simulink model "LBR7_Single_TaskComputedTorque"  (R2017b)
settings: Solver=FixedStepAuto  StartTime=0.0  StopTime=12  FixedStep=0.01  RelTol=1e-3
PreLoadFcn:
  | Preload
values from neighbouring files (symbols this model uses):
  cor_gain = -1    [Preload.m]
  joint1_gain = 1    [Preload.m]    (also in PreloadTest.m)
  joint2_gain = 1    [Preload.m]    (also in PreloadTest.m)
  joint3_gain = 1    [Preload.m]    (also in PreloadTest.m)
  joint4_gain = 1    [Preload.m]    (also in PreloadTest.m)
  joint5_gain = 1    [Preload.m]    (also in PreloadTest.m)
  joint6_gain = 1    [Preload.m]    (also in PreloadTest.m)
  joint7_gain = 1    [Preload.m]    (also in PreloadTest.m)
  kuk = SerialLink(L)    [Preload.m]    (also in PreloadTest.m)
undefined symbols (not defined in the file or in its folder): cory, gravy, inertdyn, X, Y, Z
libraries: sm_lib x77, nesl_utility x30
(part 1 of 2)
settings Model: Creator=jrv  LastModifiedBy=jrv

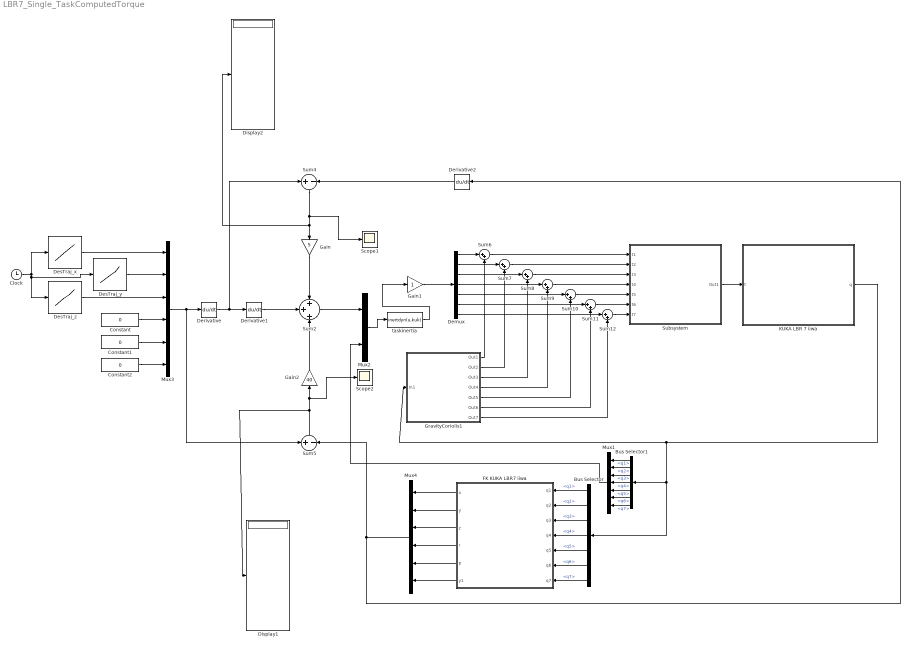
== system LBR7_Single_TaskComputedTorque ==
  Bus Selector : BusSelector  OutputSignals=q1,q2,q3,q4,q5,q6,q7
  Bus Selector1 : BusSelector  OutputSignals=q1,q2,q3,q4,q5,q6,q7
  Clock : Clock
  Constant : Constant  Value=0
  Constant1 : Constant  Value=0
  Constant2 : Constant  Value=0
  Demux : Demux  Outputs=7
  Derivative : Derivative
  Derivative1 : Derivative
  Derivative2 : Derivative
  DesTraj_x : Lookup_n-D  NumberOfTableDimensions=1  BreakpointsForDimension1=[0 5]  Table=[0.2314 0.2314]  ExtrapMethod=Clip  UseLastTableValue=on  InternalRulePriority=Speed  RndMeth=Simplest  InputSameDT=on
  DesTraj_y : Lookup_n-D  NumberOfTableDimensions=1  BreakpointsForDimension1=[0 12]  Table=[-0.2689 0.0689]  ExtrapMethod=Clip  UseLastTableValue=on  InternalRulePriority=Speed  RndMeth=Simplest  InputSameDT=on
  DesTraj_z : Lookup_n-D  NumberOfTableDimensions=1  BreakpointsForDimension1=[0 3 6 9 12]  Table=[0.9093 0.7093 0.9093 0.7093 0.9093]  InterpMethod=Cubic spline  ExtrapMethod=Clip  UseLastTableValue=on  InternalRulePriority=Speed  RndMeth=Simplest  InputSameDT=on
  Display1 : Display
  Display2 : Display
  FK KUKA LBR7 iiwa : MATLAB Function  TreatAsAtomicUnit=on
  Gain : Gain  Gain=5
  Gain1 : Gain
  Gain2 : Gain  Gain=40
  GravityCoriolis1 : Subsystem
  KUKA LBR 7 iiwa : Subsystem
  Mux1 : Mux  Inputs=7
  Mux2 : Mux  Inputs=2
  Mux3 : Mux  Inputs=6
  Mux4 : Mux  Inputs=6
  Scope1 : Scope
  Scope2 : Scope
  Subsystem : Subsystem
  Sum{6..12} (7 alike) : Sum  Inputs=|++
  Sum2 : Sum  Inputs=+++
  Sum4 : Sum  Inputs=+-
  Sum5 : Sum  Inputs=+-
  taskinertia : MATLABFcn  MATLABFcn=inertdyn(u,kuk)
  wires:
  Subsystem/1(Out1) -> KUKA LBR 7 iiwa/1(t)
  Sum4/1 -> Scope1/1, Display2/1, Gain/1
  Sum5/1 -> Scope2/1, Gain2/1, Display1/1
  GravityCoriolis1/1(Out1) -> Sum6/2
  Sum8/1 -> Subsystem/3(t3)
  GravityCoriolis1/4(Out4) -> Sum9/2
  GravityCoriolis1/2(Out2) -> Sum7/2
  Sum9/1 -> Subsystem/4(t4)
  Sum11/1 -> Subsystem/6(t6)
  Demux/7 -> Sum12/1
  Demux/5 -> Sum10/1
  GravityCoriolis1/5(Out5) -> Sum10/2
  Sum6/1 -> Subsystem/1(t1)
  Demux/1 -> Sum6/1
  Sum10/1 -> Subsystem/5(t5)
  Demux/6 -> Sum11/1
  Demux/3 -> Sum8/1
  GravityCoriolis1/6(Out6) -> Sum11/2
  Demux/4 -> Sum9/1
  Demux/2 -> Sum7/1
  Sum7/1 -> Subsystem/2(t2)
  GravityCoriolis1/3(Out3) -> Sum8/2
  Sum12/1 -> Subsystem/7(t7)
  GravityCoriolis1/7(Out7) -> Sum12/2
  Gain/1 -> Sum2/1
  Gain2/1 -> Sum2/3
  DesTraj_x/1 -> Mux3/1
  Constant2/1 -> Mux3/6
  DesTraj_y/1 -> Mux3/2
  Constant/1 -> Mux3/4
  Clock/1 -> DesTraj_y/1, DesTraj_z/1, DesTraj_x/1
  Constant1/1 -> Mux3/5
  DesTraj_z/1 -> Mux3/3
  Mux3/1 -> Sum5/1, Derivative/1
  Derivative/1 -> Sum4/1, Derivative1/1
  Derivative1/1 -> Sum2/2
  Bus Selector/1 -> FK KUKA LBR7 iiwa/1(q1)  "<q1>"
  Bus Selector/3 -> FK KUKA LBR7 iiwa/3(q3)  "<q3>"
  Bus Selector/5 -> FK KUKA LBR7 iiwa/5(q5)  "<q5>"
  Bus Selector/6 -> FK KUKA LBR7 iiwa/6(q6)  "<q6>"
  Bus Selector/2 -> FK KUKA LBR7 iiwa/2(q2)  "<q2>"
  Bus Selector/7 -> FK KUKA LBR7 iiwa/7(q7)  "<q7>"
  Bus Selector/4 -> FK KUKA LBR7 iiwa/4(q4)  "<q4>"
  FK KUKA LBR7 iiwa/3(z) -> Mux4/3
  FK KUKA LBR7 iiwa/2(y) -> Mux4/2
  FK KUKA LBR7 iiwa/4(r) -> Mux4/4
  FK KUKA LBR7 iiwa/1(x) -> Mux4/1
  FK KUKA LBR7 iiwa/5(p) -> Mux4/5
  FK KUKA LBR7 iiwa/6(y1) -> Mux4/6
  Mux4/1 -> Sum5/2, Derivative2/1
  Mux2/1 -> taskinertia/1
  taskinertia/1 -> Gain1/1
  Sum2/1 -> Mux2/1
  Mux1/1 -> Mux2/2
  KUKA LBR 7 iiwa/1(q) -> GravityCoriolis1/1(In1), Bus Selector1/1, Bus Selector/1
  Bus Selector1/1 -> Mux1/1  "<q1>"
  Bus Selector1/2 -> Mux1/2  "<q2>"
  Bus Selector1/3 -> Mux1/3  "<q3>"
  Bus Selector1/4 -> Mux1/4  "<q4>"
  Bus Selector1/5 -> Mux1/5  "<q5>"
  Bus Selector1/6 -> Mux1/6  "<q6>"
  Bus Selector1/7 -> Mux1/7  "<q7>"
  Derivative2/1 -> Sum4/2
  Gain1/1 -> Demux/1

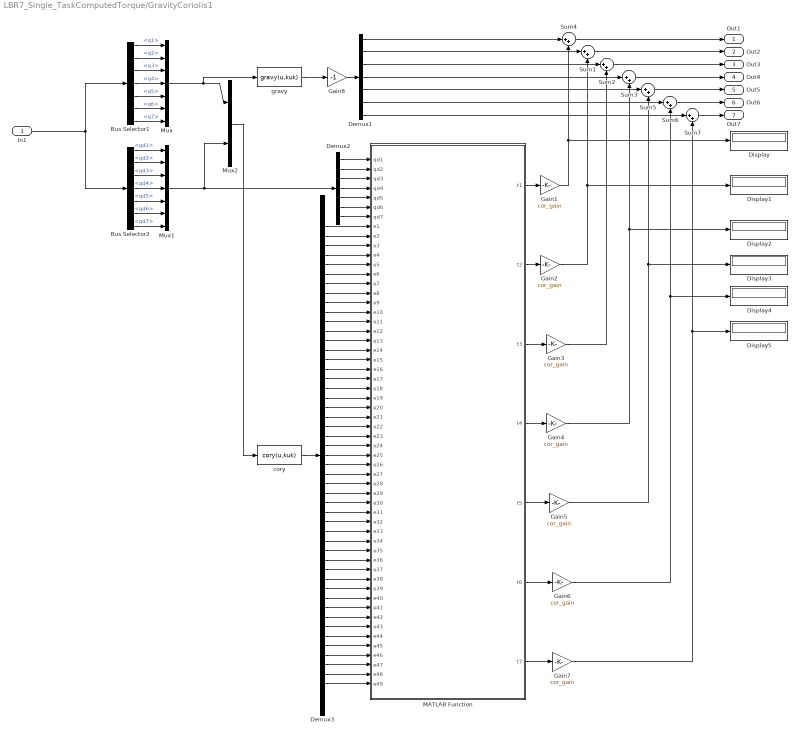
== system LBR7_Single_TaskComputedTorque/GravityCoriolis1 ==
  In1 : Inport
  Bus Selector1 : BusSelector  OutputSignals=q1,q2,q3,q4,q5,q6,q7
  Bus Selector2 : BusSelector  OutputSignals=qd1,qd2,qd3,qd4,qd5,qd6,qd7
  Demux1 : Demux  Outputs=7
  Demux2 : Demux  Outputs=7
  Demux3 : Demux  Outputs=49
  Display{,1..5} (6 alike) : Display
  Gain{1..7} (7 alike) : Gain  Gain=cor_gain
  Gain8 : Gain  Gain=-1
  MATLAB Function : MATLAB Function  TreatAsAtomicUnit=on
  Mux : Mux  Inputs=7
  Mux1 : Mux  Inputs=7
  Mux2 : Mux  Inputs=2
  Sum{1..7} (7 alike) : Sum  Inputs=|++
  cory : MATLABFcn  MATLABFcn=cory(u,kuk)
  gravy : MATLABFcn  MATLABFcn=gravy(u,kuk)
  Out1 : Outport
  Out2 : Outport  Port=2
  Out3 : Outport  Port=3
  Out4 : Outport  Port=4
  Out5 : Outport  Port=5
  Out6 : Outport  Port=6
  Out7 : Outport  Port=7
  wires:
  Demux2/1 -> MATLAB Function/1(qd1)
  Mux1/1 -> Mux2/2, Demux2/1
  Demux3/16 -> MATLAB Function/23(e16)
  Mux/1 -> gravy/1, Mux2/1
  Bus Selector1/2 -> Mux/2  "<q2>"
  Demux3/29 -> MATLAB Function/36(e29)
  Demux3/35 -> MATLAB Function/42(e35)
  Demux3/15 -> MATLAB Function/22(e15)
  Demux3/22 -> MATLAB Function/29(e22)
  Demux3/9 -> MATLAB Function/16(e9)
  Bus Selector1/3 -> Mux/3  "<q3>"
  Demux3/11 -> MATLAB Function/18(e11)
  Bus Selector1/7 -> Mux/7  "<q7>"
  Demux3/42 -> MATLAB Function/49(e42)
  Demux3/43 -> MATLAB Function/50(e43)
  Bus Selector1/1 -> Mux/1  "<q1>"
  Bus Selector1/5 -> Mux/5  "<q5>"
  Demux3/24 -> MATLAB Function/31(e24)
  Bus Selector1/6 -> Mux/6  "<q6>"
  Demux3/26 -> MATLAB Function/33(e26)
  Bus Selector1/4 -> Mux/4  "<q4>"
  Demux3/14 -> MATLAB Function/21(e14)
  Demux3/19 -> MATLAB Function/26(e19)
  Demux3/4 -> MATLAB Function/11(e4)
  Bus Selector2/4 -> Mux1/4  "<qd4>"
  cory/1 -> Demux3/1
  Demux3/23 -> MATLAB Function/30(e23)
  Demux2/3 -> MATLAB Function/3(qd3)
  Demux3/31 -> MATLAB Function/38(e31)
  Demux2/4 -> MATLAB Function/4(qd4)
  Demux3/17 -> MATLAB Function/24(e17)
  Demux2/5 -> MATLAB Function/5(qd5)
  Demux3/3 -> MATLAB Function/10(e3)
  Demux3/20 -> MATLAB Function/27(e20)
  Demux3/36 -> MATLAB Function/43(e36)
  In1/1 -> Bus Selector2/1, Bus Selector1/1
  Bus Selector2/6 -> Mux1/6  "<qd6>"
  Demux3/40 -> MATLAB Function/47(e40)
  Demux3/8 -> MATLAB Function/15(e8)
  Demux3/45 -> MATLAB Function/52(e45)
  Demux3/28 -> MATLAB Function/35(e28)
  Demux3/41 -> MATLAB Function/48(e41)
  Bus Selector2/5 -> Mux1/5  "<qd5>"
  Demux3/49 -> MATLAB Function/56(e49)
  Demux3/27 -> MATLAB Function/34(e27)
  Demux3/13 -> MATLAB Function/20(e13)
  Demux3/6 -> MATLAB Function/13(e6)
  Demux3/30 -> MATLAB Function/37(e30)
  Demux2/7 -> MATLAB Function/7(qd7)
  Demux3/25 -> MATLAB Function/32(e25)
  Demux2/2 -> MATLAB Function/2(qd2)
  Demux3/5 -> MATLAB Function/12(e5)
  Bus Selector2/7 -> Mux1/7  "<qd7>"
  Demux3/7 -> MATLAB Function/14(e7)
  Bus Selector2/3 -> Mux1/3  "<qd3>"
  Mux2/1 -> cory/1
  Demux1/1 -> Sum4/1
  Demux3/1 -> MATLAB Function/8(e1)
  Demux3/33 -> MATLAB Function/40(e33)
  Demux3/12 -> MATLAB Function/19(e12)
  Bus Selector2/1 -> Mux1/1  "<qd1>"
  Demux1/4 -> Sum3/1
  Demux3/48 -> MATLAB Function/55(e48)
  Demux3/32 -> MATLAB Function/39(e32)
  Demux3/34 -> MATLAB Function/41(e34)
  Demux3/47 -> MATLAB Function/54(e47)
  Bus Selector2/2 -> Mux1/2  "<qd2>"
  Demux2/6 -> MATLAB Function/6(qd6)
  Sum7/1 -> Out7/1
  Demux3/39 -> MATLAB Function/46(e39)
  Sum3/1 -> Out4/1
  Sum6/1 -> Out6/1
  Demux1/3 -> Sum2/1
  Demux3/21 -> MATLAB Function/28(e21)
  Sum1/1 -> Out2/1
  Demux1/2 -> Sum1/1
  Sum4/1 -> Out1/1
  Demux1/5 -> Sum5/1
  Demux3/2 -> MATLAB Function/9(e2)
  Demux3/18 -> MATLAB Function/25(e18)
  Demux3/38 -> MATLAB Function/45(e38)
  Demux3/46 -> MATLAB Function/53(e46)
  Sum5/1 -> Out5/1
  Demux3/37 -> MATLAB Function/44(e37)
  Demux3/44 -> MATLAB Function/51(e44)
  Sum2/1 -> Out3/1
  Demux3/10 -> MATLAB Function/17(e10)
  Gain2/1 -> Display1/1, Sum1/2
  Gain4/1 -> Display2/1, Sum3/2
  Gain6/1 -> Display4/1, Sum6/2
  Gain3/1 -> Sum2/2
  Gain5/1 -> Display3/1, Sum5/2
  Demux1/7 -> Sum7/1
  Gain7/1 -> Display5/1, Sum7/2
  Gain8/1 -> Demux1/1
  Demux1/6 -> Sum6/1
  gravy/1 -> Gain8/1
  Gain1/1 -> Display/1, Sum4/2
  MATLAB Function/1(t1) -> Gain1/1
  MATLAB Function/2(t2) -> Gain2/1
  MATLAB Function/3(t3) -> Gain3/1
  MATLAB Function/4(t4) -> Gain4/1
  MATLAB Function/5(t5) -> Gain5/1
  MATLAB Function/6(t6) -> Gain6/1
  MATLAB Function/7(t7) -> Gain7/1

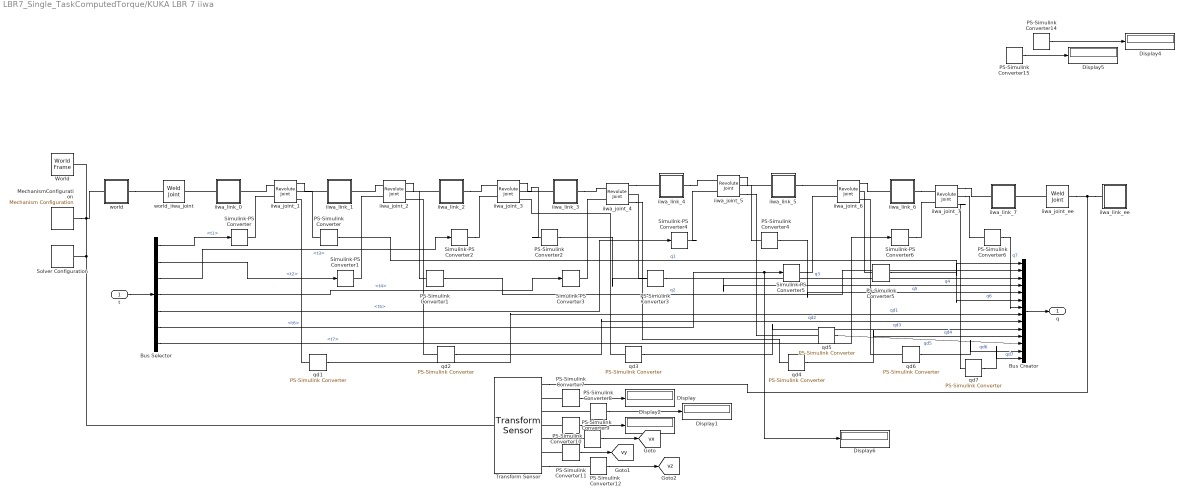
== system LBR7_Single_TaskComputedTorque/KUKA LBR 7 iiwa ==
  t : Inport
  Bus Creator : BusCreator  Inputs=14
  Bus Selector : BusSelector  OutputSignals=t1,t2,t3,t4,t5,t6,t7
  Display{,1..2,4..6} (6 alike) : Display
  MechanismConfiguration : sm_lib/Utilities/Mechanism Configuration  UniformGravity=Constant  GravityVector=[0 0 -9.81]  GravityUnits=m/s^2  LinearizationDelta=0.001
  PS-Simulink Converter{,1..6} (7 alike) : nesl_utility/PS-Simulink Converter  PhysicalDomain=network_engine_domain  SubClassName=ps_output  LeftPortType=input  RightPortType=output  PseudoPeriodic=off  Frequencies=[]  Unit=rad  AffineConversion=off
  PS-Simulink Converter10 : nesl_utility/PS-Simulink Converter  PhysicalDomain=network_engine_domain  SubClassName=ps_output  LeftPortType=input  RightPortType=output  PseudoPeriodic=off  Frequencies=[]  Unit=m/s  AffineConversion=off
  PS-Simulink Converter11 : nesl_utility/PS-Simulink Converter  PhysicalDomain=network_engine_domain  SubClassName=ps_output  LeftPortType=input  RightPortType=output  PseudoPeriodic=off  Frequencies=[]  Unit=m/s  AffineConversion=off
  PS-Simulink Converter12 : nesl_utility/PS-Simulink Converter  PhysicalDomain=network_engine_domain  SubClassName=ps_output  LeftPortType=input  RightPortType=output  PseudoPeriodic=off  Frequencies=[]  Unit=m/s  AffineConversion=off
  PS-Simulink Converter{7..9,14..15} (5 alike) : nesl_utility/PS-Simulink Converter  PhysicalDomain=network_engine_domain  SubClassName=ps_output  LeftPortType=input  RightPortType=output  PseudoPeriodic=off  Frequencies=[]  Unit=1  AffineConversion=off
  Simulink-PS Converter{,1..6} (7 alike) : nesl_utility/Simulink-PS Converter  PhysicalDomain=network_engine_domain  SubClassName=ps_input  LeftPortType=input  RightPortType=output  PseudoPeriodic=off  Frequencies=[]  NoiseDistribution=none  NoiseParameters=[]  Unit=N*m  AffineConversion=off  FilteringAndDerivatives=provide  SimscapeFilterOrder=1  InputFilterTimeConstant=0.001  UdotUserProvided=0
  Solver Configuration : nesl_utility/Solver Configuration  PhysicalDomain=network_engine_domain  SubClassName=solver  LeftPortType=input  RightPortType=generic  Accelerate=off  Tones=[]  Harmonics=[]  SimulateNoise=off  Profile=off  UseLocalSampling=off  EnableSwitchedLinearOptims=on  FrequencyDomain=off  UseCCode=off  RelTol=0.001  AbsTol=1e-06  MinStep=1e-09  ToWorkspace=off  RevertToSquareIcSolve=off  NumHomotopyIterations=100  PhasorMode=off  PhasorModeNumHarmonics=1  DoDC=off  ResidualTolerance=1e-09  UseLocalSolver=off  LocalSolverChoice=NE_BACKWARD_EULER_ADVANCER  LocalSolverSampleTime=0.001  DoFixedCost=off  MaxNonlinIter=3  MaxModeIter=2  LinearAlgebra=Sparse  DelaysMemoryBudget=1024  AutomaticFiltering=on  FilteringTimeConstant=0.001
  Transform Sensor : sm_lib/Frames and Transforms/Transform Sensor  MeasurementFrame=World  SenseAngle=off  SenseAxis=off  SenseAngle1=off  SenseAngle2=off  SenseAngle3=off  SenseQ=off  SenseR=off  SenseOmegaX=off  SenseOmegaY=off  SenseOmegaZ=off  SenseOmega1=off  SenseOmega2=off  SenseOmega3=off  SenseQDot=off  SenseRDot=off  SenseAlphaX=off  SenseAlphaY=off  SenseAlphaZ=off  SenseAlpha1=off  SenseAlpha2=off  SenseAlpha3=off  SenseQDDot=off  SenseRDDot=off  SenseX=on  SenseY=on  SenseZ=on  SenseRad=off  SenseAzim=off  SenseDist=off  SenseInc=off  SenseXDot=on  SenseYDot=on  SenseZDot=on  SenseRadDot=off  SenseAzimDot=off  SenseDistDot=off  SenseIncDot=off  SenseXDDot=off  SenseYDDot=off  SenseZDDot=off  SenseRadDDot=off  SenseAzimDDot=off  SenseDistDDot=off  SenseIncDDot=off
  World : sm_lib/Frames and Transforms/World Frame
  iiwa_joint_1 : sm_lib/Joints/Revolute Joint  SenseConstraintForce=off  SenseConstraintForceX=off  SenseConstraintForceY=off  SenseConstraintForceZ=off  SenseConstraintTorque=off  SenseConstraintTorqueX=off  SenseConstraintTorqueY=off  SenseConstraintTorqueZ=off  SenseTotalForce=off  SenseTotalForceX=off  SenseTotalForceY=off  SenseTotalForceZ=off  SenseTotalTorque=off  SenseTotalTorqueX=off  SenseTotalTorqueY=off  SenseTotalTorqueZ=off  CompositeWrenchDir=FollowerOnBase  CompositeWrenchFrame=BaseFrame  EquilibriumPosition=0  EquilibriumPositionUnits=deg  SpringStiffness=0  SpringStiffnessUnits=N*m/deg  DampingCoefficient=joint1_damping  DampingCoefficientUnits=m^2*kg/s/rad  TorqueActuationMode=InputTorque  MotionActuationMode=ComputedMotion  SensePosition=on  SenseVelocity=on  SenseAcceleration=off  SenseTorqueForce=off  PositionTargetSpecify=on  PositionTargetPriority=High  PositionTargetValue=joint1_initial_deg  PositionTargetValueUnits=deg  VelocityTargetSpecify=off  VelocityTargetPriority=High  VelocityTargetValue=0  VelocityTargetValueUnits=deg/s
  iiwa_joint_2 : sm_lib/Joints/Revolute Joint  SenseConstraintForce=off  SenseConstraintForceX=off  SenseConstraintForceY=off  SenseConstraintForceZ=off  SenseConstraintTorque=off  SenseConstraintTorqueX=off  SenseConstraintTorqueY=off  SenseConstraintTorqueZ=off  SenseTotalForce=off  SenseTotalForceX=off  SenseTotalForceY=off  SenseTotalForceZ=off  SenseTotalTorque=off  SenseTotalTorqueX=off  SenseTotalTorqueY=off  SenseTotalTorqueZ=off  CompositeWrenchDir=FollowerOnBase  CompositeWrenchFrame=BaseFrame  EquilibriumPosition=0  EquilibriumPositionUnits=deg  SpringStiffness=0  SpringStiffnessUnits=N*m/deg  DampingCoefficient=joint2_damping  DampingCoefficientUnits=m^2*kg/s/rad  TorqueActuationMode=InputTorque  MotionActuationMode=ComputedMotion  SensePosition=on  SenseVelocity=on  SenseAcceleration=off  SenseTorqueForce=off  PositionTargetSpecify=on  PositionTargetPriority=High  PositionTargetValue=joint2_initial_deg  PositionTargetValueUnits=deg  VelocityTargetSpecify=off  VelocityTargetPriority=High  VelocityTargetValue=0  VelocityTargetValueUnits=deg/s
  iiwa_joint_3 : sm_lib/Joints/Revolute Joint  SenseConstraintForce=off  SenseConstraintForceX=off  SenseConstraintForceY=off  SenseConstraintForceZ=off  SenseConstraintTorque=off  SenseConstraintTorqueX=off  SenseConstraintTorqueY=off  SenseConstraintTorqueZ=off  SenseTotalForce=off  SenseTotalForceX=off  SenseTotalForceY=off  SenseTotalForceZ=off  SenseTotalTorque=off  SenseTotalTorqueX=off  SenseTotalTorqueY=off  SenseTotalTorqueZ=off  CompositeWrenchDir=FollowerOnBase  CompositeWrenchFrame=BaseFrame  EquilibriumPosition=0  EquilibriumPositionUnits=deg  SpringStiffness=0  SpringStiffnessUnits=N*m/deg  DampingCoefficient=joint3_damping  DampingCoefficientUnits=m^2*kg/s/rad  TorqueActuationMode=InputTorque  MotionActuationMode=ComputedMotion  SensePosition=on  SenseVelocity=on  SenseAcceleration=off  SenseTorqueForce=off  PositionTargetSpecify=on  PositionTargetPriority=High  PositionTargetValue=joint3_initial_deg  PositionTargetValueUnits=deg  VelocityTargetSpecify=off  VelocityTargetPriority=High  VelocityTargetValue=0  VelocityTargetValueUnits=deg/s
  iiwa_joint_4 : sm_lib/Joints/Revolute Joint  SenseConstraintForce=off  SenseConstraintForceX=off  SenseConstraintForceY=off  SenseConstraintForceZ=off  SenseConstraintTorque=off  SenseConstraintTorqueX=off  SenseConstraintTorqueY=off  SenseConstraintTorqueZ=off  SenseTotalForce=off  SenseTotalForceX=off  SenseTotalForceY=off  SenseTotalForceZ=off  SenseTotalTorque=off  SenseTotalTorqueX=off  SenseTotalTorqueY=off  SenseTotalTorqueZ=off  CompositeWrenchDir=FollowerOnBase  CompositeWrenchFrame=BaseFrame  EquilibriumPosition=0  EquilibriumPositionUnits=deg  SpringStiffness=0  SpringStiffnessUnits=N*m/deg  DampingCoefficient=joint4_damping  DampingCoefficientUnits=m^2*kg/s/rad  TorqueActuationMode=InputTorque  MotionActuationMode=ComputedMotion  SensePosition=on  SenseVelocity=on  SenseAcceleration=off  SenseTorqueForce=off  PositionTargetSpecify=on  PositionTargetPriority=High  PositionTargetValue=joint4_initial_deg  PositionTargetValueUnits=deg  VelocityTargetSpecify=off  VelocityTargetPriority=High  VelocityTargetValue=0  VelocityTargetValueUnits=deg/s
  iiwa_joint_5 : sm_lib/Joints/Revolute Joint  SenseConstraintForce=off  SenseConstraintForceX=off  SenseConstraintForceY=off  SenseConstraintForceZ=off  SenseConstraintTorque=off  SenseConstraintTorqueX=off  SenseConstraintTorqueY=off  SenseConstraintTorqueZ=off  SenseTotalForce=off  SenseTotalForceX=off  SenseTotalForceY=off  SenseTotalForceZ=off  SenseTotalTorque=off  SenseTotalTorqueX=off  SenseTotalTorqueY=off  SenseTotalTorqueZ=off  CompositeWrenchDir=FollowerOnBase  CompositeWrenchFrame=BaseFrame  EquilibriumPosition=0  EquilibriumPositionUnits=deg  SpringStiffness=0  SpringStiffnessUnits=N*m/deg  DampingCoefficient=joint5_damping  DampingCoefficientUnits=m^2*kg/s/rad  TorqueActuationMode=InputTorque  MotionActuationMode=ComputedMotion  SensePosition=on  SenseVelocity=on  SenseAcceleration=off  SenseTorqueForce=off  PositionTargetSpecify=on  PositionTargetPriority=High  PositionTargetValue=joint5_initial_deg  PositionTargetValueUnits=deg  VelocityTargetSpecify=off  VelocityTargetPriority=High  VelocityTargetValue=0  VelocityTargetValueUnits=deg/s
  iiwa_joint_6 : sm_lib/Joints/Revolute Joint  SenseConstraintForce=off  SenseConstraintForceX=off  SenseConstraintForceY=off  SenseConstraintForceZ=off  SenseConstraintTorque=off  SenseConstraintTorqueX=off  SenseConstraintTorqueY=off  SenseConstraintTorqueZ=off  SenseTotalForce=off  SenseTotalForceX=off  SenseTotalForceY=off  SenseTotalForceZ=off  SenseTotalTorque=off  SenseTotalTorqueX=off  SenseTotalTorqueY=off  SenseTotalTorqueZ=off  CompositeWrenchDir=FollowerOnBase  CompositeWrenchFrame=BaseFrame  EquilibriumPosition=0  EquilibriumPositionUnits=deg  SpringStiffness=0  SpringStiffnessUnits=N*m/deg  DampingCoefficient=joint6_damping  DampingCoefficientUnits=m^2*kg/s/rad  TorqueActuationMode=InputTorque  MotionActuationMode=ComputedMotion  SensePosition=on  SenseVelocity=on  SenseAcceleration=off  SenseTorqueForce=off  PositionTargetSpecify=on  PositionTargetPriority=High  PositionTargetValue=joint6_initial_deg  PositionTargetValueUnits=deg  VelocityTargetSpecify=off  VelocityTargetPriority=High  VelocityTargetValue=0  VelocityTargetValueUnits=deg/s
  iiwa_joint_7 : sm_lib/Joints/Revolute Joint  SenseConstraintForce=off  SenseConstraintForceX=off  SenseConstraintForceY=off  SenseConstraintForceZ=off  SenseConstraintTorque=off  SenseConstraintTorqueX=off  SenseConstraintTorqueY=off  SenseConstraintTorqueZ=off  SenseTotalForce=off  SenseTotalForceX=off  SenseTotalForceY=off  SenseTotalForceZ=off  SenseTotalTorque=off  SenseTotalTorqueX=off  SenseTotalTorqueY=off  SenseTotalTorqueZ=off  CompositeWrenchDir=FollowerOnBase  CompositeWrenchFrame=BaseFrame  EquilibriumPosition=0  EquilibriumPositionUnits=deg  SpringStiffness=0  SpringStiffnessUnits=N*m/deg  DampingCoefficient=joint7_damping  DampingCoefficientUnits=m^2*kg/s/rad  TorqueActuationMode=InputTorque  MotionActuationMode=ComputedMotion  SensePosition=on  SenseVelocity=on  SenseAcceleration=off  SenseTorqueForce=off  PositionTargetSpecify=on  PositionTargetPriority=High  PositionTargetValue=joint7_initial_deg  PositionTargetValueUnits=deg  VelocityTargetSpecify=off  VelocityTargetPriority=High  VelocityTargetValue=0  VelocityTargetValueUnits=deg/s
  iiwa_joint_ee : sm_lib/Joints/Weld Joint  SenseConstraintForce=off  SenseConstraintForceX=off  SenseConstraintForceY=off  SenseConstraintForceZ=off  SenseConstraintTorque=off  SenseConstraintTorqueX=off  SenseConstraintTorqueY=off  SenseConstraintTorqueZ=off  SenseTotalForce=off  SenseTotalForceX=off  SenseTotalForceY=off  SenseTotalForceZ=off  SenseTotalTorque=off  SenseTotalTorqueX=off  SenseTotalTorqueY=off  SenseTotalTorqueZ=off  CompositeWrenchDir=FollowerOnBase  CompositeWrenchFrame=BaseFrame
  iiwa_link_0 : Subsystem
  iiwa_link_1 : Subsystem
  iiwa_link_2 : Subsystem
  iiwa_link_3 : Subsystem
  iiwa_link_4 : Subsystem
  iiwa_link_5 : Subsystem
  iiwa_link_6 : Subsystem
  iiwa_link_7 : Subsystem
  iiwa_link_ee : Subsystem
  qd{1..7} (7 alike) : nesl_utility/PS-Simulink Converter  PhysicalDomain=network_engine_domain  SubClassName=ps_output  LeftPortType=input  RightPortType=output  PseudoPeriodic=off  Frequencies=[]  Unit=rad/s  AffineConversion=off
  world : Subsystem
  world_iiwa_joint : sm_lib/Joints/Weld Joint  SenseConstraintForce=off  SenseConstraintForceX=off  SenseConstraintForceY=off  SenseConstraintForceZ=off  SenseConstraintTorque=off  SenseConstraintTorqueX=off  SenseConstraintTorqueY=off  SenseConstraintTorqueZ=off  SenseTotalForce=off  SenseTotalForceX=off  SenseTotalForceY=off  SenseTotalForceZ=off  SenseTotalTorque=off  SenseTotalTorqueX=off  SenseTotalTorqueY=off  SenseTotalTorqueZ=off  CompositeWrenchDir=FollowerOnBase  CompositeWrenchFrame=BaseFrame
  q : Outport
  tag scope: vx=global, vy=global, vz=global
  wires:
  PS-Simulink Converter7/1 -> Display/1
  PS-Simulink Converter9/1 -> Display2/1
  PS-Simulink Converter8/1 -> Display1/1
  PS-Simulink Converter/1 -> Bus Creator/1  "q1"
  PS-Simulink Converter1/1 -> Bus Creator/2  "q2"
  PS-Simulink Converter2/1 -> Bus Creator/3  "q3"
  PS-Simulink Converter3/1 -> Bus Creator/4  "q4"
  PS-Simulink Converter4/1 -> Bus Creator/5  "q5"
  PS-Simulink Converter5/1 -> Bus Creator/6  "q6"
  PS-Simulink Converter6/1 -> Bus Creator/7  "q7"
  Bus Creator/1 -> q/1
  t/1 -> Bus Selector/1
  Bus Selector/1 -> Simulink-PS Converter/1  "<t1>"
  Bus Selector/2 -> Simulink-PS Converter1/1  "<t2>"
  Bus Selector/3 -> Simulink-PS Converter2/1  "<t3>"
  Bus Selector/4 -> Simulink-PS Converter3/1  "<t4>"
  Bus Selector/5 -> Simulink-PS Converter4/1  "<t5>"
  Bus Selector/6 -> Display6/1, Simulink-PS Converter5/1  "<t6>"
  Bus Selector/7 -> Simulink-PS Converter6/1  "<t7>"
  qd1/1 -> Bus Creator/8  "qd1"
  qd2/1 -> Bus Creator/9  "qd2"
  qd3/1 -> Bus Creator/10  "qd3"
  qd4/1 -> Bus Creator/11  "qd4"
  qd5/1 -> Bus Creator/12  "qd5"
  qd6/1 -> Bus Creator/13  "qd6"
  qd7/1 -> Bus Creator/14  "qd7"
  PS-Simulink Converter10/1 -> [vx]
  PS-Simulink Converter11/1 -> [vy]
  PS-Simulink Converter12/1 -> [vz]
  PS-Simulink Converter14/1 -> Display4/1
  PS-Simulink Converter15/1 -> Display5/1
  connections:
  Simulink-PS Converter/RConn1 -- iiwa_joint_1/LConn2
  PS-Simulink Converter/LConn1 -- iiwa_joint_1/RConn2
  iiwa_joint_2/LConn2 -- Simulink-PS Converter1/RConn1
  iiwa_joint_2/RConn2 -- PS-Simulink Converter1/LConn1
  iiwa_joint_1/LConn1 -- iiwa_link_0/RConn1
  iiwa_joint_2/RConn1 -- iiwa_link_2/LConn1
  iiwa_link_0/LConn1 -- world_iiwa_joint/RConn1
  world/RConn1 -- world_iiwa_joint/LConn1
  World/RConn1 -- Transform Sensor/LConn1 -- Solver Configuration/RConn1 -- MechanismConfiguration/RConn1 -- world/LConn1
  iiwa_joint_2/LConn1 -- iiwa_link_1/RConn1
  iiwa_joint_1/RConn1 -- iiwa_link_1/LConn1
  PS-Simulink Converter9/LConn1 -- Transform Sensor/RConn4
  PS-Simulink Converter8/LConn1 -- Transform Sensor/RConn3
  PS-Simulink Converter7/LConn1 -- Transform Sensor/RConn2
  qd1/LConn1 -- iiwa_joint_1/RConn3
  qd2/LConn1 -- iiwa_joint_2/RConn3
  PS-Simulink Converter10/LConn1 -- Transform Sensor/RConn5
  PS-Simulink Converter11/LConn1 -- Transform Sensor/RConn6
  Transform Sensor/RConn7 -- PS-Simulink Converter12/LConn1
  Simulink-PS Converter2/RConn1 -- iiwa_joint_3/LConn2
  iiwa_link_2/RConn1 -- iiwa_joint_3/LConn1
  PS-Simulink Converter2/LConn1 -- iiwa_joint_3/RConn2
  iiwa_joint_3/RConn1 -- iiwa_link_3/LConn1
  qd3/LConn1 -- iiwa_joint_3/RConn3
  iiwa_link_3/RConn1 -- iiwa_joint_4/LConn1
  iiwa_joint_4/RConn1 -- iiwa_link_4/LConn1
  Simulink-PS Converter3/RConn1 -- iiwa_joint_4/LConn2
  PS-Simulink Converter3/LConn1 -- iiwa_joint_4/RConn2
  iiwa_joint_5/RConn1 -- iiwa_link_5/LConn1
  iiwa_link_4/RConn1 -- iiwa_joint_5/LConn1
  Simulink-PS Converter4/RConn1 -- iiwa_joint_5/LConn2
  iiwa_joint_5/RConn2 -- PS-Simulink Converter4/LConn1
  iiwa_joint_5/RConn3 -- qd5/LConn1
  iiwa_joint_4/RConn3 -- qd4/LConn1
  qd6/LConn1 -- iiwa_joint_6/RConn3
  PS-Simulink Converter5/LConn1 -- iiwa_joint_6/RConn2
  iiwa_link_5/RConn1 -- iiwa_joint_6/LConn1
  iiwa_joint_6/RConn1 -- iiwa_link_6/LConn1
  Simulink-PS Converter5/RConn1 -- iiwa_joint_6/LConn2
  iiwa_link_ee/LConn1 -- Transform Sensor/RConn1 -- iiwa_joint_ee/RConn1
  iiwa_joint_ee/LConn1 -- iiwa_link_7/RConn1
  iiwa_joint_7/RConn3 -- qd7/LConn1
  iiwa_joint_7/RConn2 -- PS-Simulink Converter6/LConn1
  iiwa_joint_7/RConn1 -- iiwa_link_7/LConn1
  Simulink-PS Converter6/RConn1 -- iiwa_joint_7/LConn2
  iiwa_link_6/RConn1 -- iiwa_joint_7/LConn1

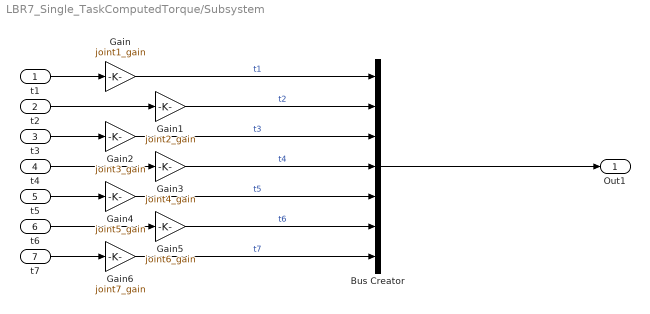
== system LBR7_Single_TaskComputedTorque/Subsystem ==
  t1 : Inport
  t2 : Inport  Port=2
  t3 : Inport  Port=3
  t4 : Inport  Port=4
  t5 : Inport  Port=5
  t6 : Inport  Port=6
  t7 : Inport  Port=7
  Bus Creator : BusCreator  Inputs=7
  Gain : Gain  Gain=joint1_gain
  Gain1 : Gain  Gain=joint2_gain
  Gain2 : Gain  Gain=joint3_gain
  Gain3 : Gain  Gain=joint4_gain
  Gain4 : Gain  Gain=joint5_gain
  Gain5 : Gain  Gain=joint6_gain
  Gain6 : Gain  Gain=joint7_gain
  Out1 : Outport
  wires:
  Bus Creator/1 -> Out1/1
  Gain/1 -> Bus Creator/1  "t1"
  Gain1/1 -> Bus Creator/2  "t2"
  Gain2/1 -> Bus Creator/3  "t3"
  Gain3/1 -> Bus Creator/4  "t4"
  Gain4/1 -> Bus Creator/5  "t5"
  Gain5/1 -> Bus Creator/6  "t6"
  Gain6/1 -> Bus Creator/7  "t7"
  t1/1 -> Gain/1
  t2/1 -> Gain1/1
  t3/1 -> Gain2/1
  t4/1 -> Gain3/1
  t5/1 -> Gain4/1
  t6/1 -> Gain5/1
  t7/1 -> Gain6/1

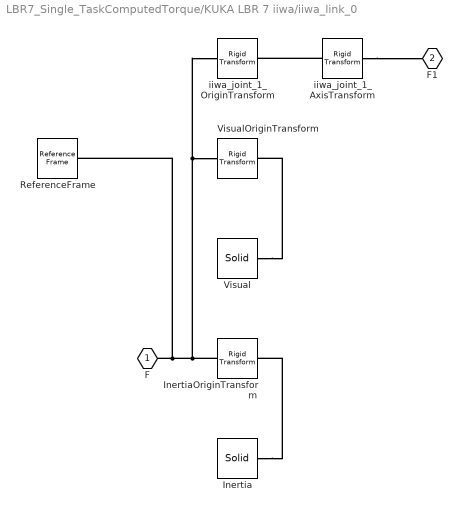
== system LBR7_Single_TaskComputedTorque/KUKA LBR 7 iiwa/iiwa_link_0 ==
  Inertia : sm_lib/Body Elements/Solid  InertiaType=Custom  Mass=5  MassUnits=kg  CenterOfMass=[0, 0, 0]  CenterOfMassUnits=m  MomentsOfInertia=[0.05, 0.06, 0.03]  MomentsOfInertiaUnits=kg*m^2  ProductsOfInertia=[0, 0, 0]  ProductsOfInertiaUnits=kg*m^2  DensityBased=on  Density=1000  DensityUnits=kg/m^3  DoExposeReferenceFrame=on  SerializedFrames=<Frames/>  GraphicType=None  MarkerShape=Sphere  MarkerSize=10  GraphicVisPropType=SimpleVisualProperties  GraphicDiffuseColor=[0.5 0.5 0.5]  GraphicSpecularColor=[0.5 0.5 0.5 1.0]  GraphicAmbientColor=[0.15 0.15 0.15 1.0]  GraphicEmissiveColor=[0.0 0.0 0.0 1.0]  GraphicShininess=75  GraphicOpacity=1.0  GeometryShape=Sphere  RectangleSize=[1 1]  RectangleSizeUnits=m  BrickDimensions=[1 1 1]  BrickDimensionUnits=m  CylinderRadius=1  CylinderRadiusUnits=m  CylinderLength=1  CylinderLengthUnits=m  SphereRadius=1  SphereRadiusUnits=m  EllipsoidRadii=[1 1 1]  EllipsoidRadiiUnits=m  ExtrusionCrossSection=[1 1; -1 1; -1 -1; 1 -1]  ExtrusionCrossSectionUnits=m  ExtrusionLength=1  ExtrusionLengthUnits=m  PolygonNumSides=3  PolygonOuterRadius=1  PolygonOuterRadiusUnits=m  ExtGeomFileType=STEP  ExtGeomFileUnits=m  RevolutionCrossSection=[1 1; 1 -1; 2 -1; 2 1]  RevolutionCrossSectionUnits=m  RevolutionExtent=Full  RevolutionAngle=180  RevolutionAngleUnits=deg
  InertiaOriginTransform : sm_lib/Frames and Transforms/Rigid Transform  TranslationMethod=Cartesian  TranslationStandardOffset=0  TranslationLengthUnit=m  TranslationStandardAxis=+Z  TranslationCartesianOffset=[-0.1, 0, 0.07000000000000001]  TranslationROffset=0  TranslationROffsetUnits=m  TranslationZOffset=0  TranslationZOffsetUnits=m  TranslationThetaOffset=0  TranslationThetaOffsetUnits=deg  RotationMethod=RotationSequence  RotationAngleUnits=deg  RotationStandardAxis=+Z  RotationAngle=0.0  RotationArbitraryAxis=[0 0 1]  FollAlignAxisA=+X  BaseAlignAxisA=+Y  FollAlignAxisB=+Y  BaseAlignAxisB=+Z  RotationSequenceAxes=BaseAxes  RotationSequence=XYZ  RotationSequenceAngles=[0, 0, 0]  RotationSequenceAnglesUnits=rad  RotationMatrix=[1 0 0; 0 1 0; 0 0 1]
  ReferenceFrame : sm_lib/Frames and Transforms/Reference Frame
  Visual : sm_lib/Body Elements/Solid  InertiaType=Custom  Mass=0  MassUnits=kg  CenterOfMass=[0, 0, 0]  CenterOfMassUnits=m  MomentsOfInertia=[0, 0, 0]  MomentsOfInertiaUnits=kg*m^2  ProductsOfInertia=[0, 0, 0]  ProductsOfInertiaUnits=kg*m^2  DensityBased=on  Density=1000  DensityUnits=kg/m^3  DoExposeReferenceFrame=on  SerializedFrames=<Frames/>  GraphicType=FromGeometry  MarkerShape=Sphere  MarkerSize=10  GraphicVisPropType=SimpleVisualProperties  GraphicDiffuseColor=[0.4, 0.4, 0.4]  GraphicSpecularColor=[0.5 0.5 0.5 1.0]  GraphicAmbientColor=[0.15 0.15 0.15 1.0]  GraphicEmissiveColor=[0.0 0.0 0.0 1.0]  GraphicShininess=75  GraphicOpacity=1  GeometryShape=FromFile  RectangleSize=[1 1]  RectangleSizeUnits=m  BrickDimensions=[1 1 1]  BrickDimensionUnits=m  CylinderRadius=1  CylinderRadiusUnits=m  CylinderLength=1  CylinderLengthUnits=m  SphereRadius=1  SphereRadiusUnits=m  EllipsoidRadii=[1 1 1]  EllipsoidRadiiUnits=m  ExtrusionCrossSection=[1 1; -1 1; -1 -1; 1 -1]  ExtrusionCrossSectionUnits=m  ExtrusionLength=1  ExtrusionLengthUnits=m  PolygonNumSides=3  PolygonOuterRadius=1  PolygonOuterRadiusUnits=m  ExtGeomFileType=STL  ExtGeomFileName=base_link.stl  ExtGeomFileUnits=m  RevolutionCrossSection=[1 1; 1 -1; 2 -1; 2 1]  RevolutionCrossSectionUnits=m  RevolutionExtent=Full  RevolutionAngle=180  RevolutionAngleUnits=deg
  VisualOriginTransform : sm_lib/Frames and Transforms/Rigid Transform  TranslationMethod=Cartesian  TranslationStandardOffset=0  TranslationLengthUnit=m  TranslationStandardAxis=+Z  TranslationCartesianOffset=[0, 0, 0]  TranslationROffset=0  TranslationROffsetUnits=m  TranslationZOffset=0  TranslationZOffsetUnits=m  TranslationThetaOffset=0  TranslationThetaOffsetUnits=deg  RotationMethod=RotationSequence  RotationAngleUnits=deg  RotationStandardAxis=+Z  RotationAngle=0.0  RotationArbitraryAxis=[0 0 1]  FollAlignAxisA=+X  BaseAlignAxisA=+Y  FollAlignAxisB=+Y  BaseAlignAxisB=+Z  RotationSequenceAxes=BaseAxes  RotationSequence=XYZ  RotationSequenceAngles=[0, 0, 0]  RotationSequenceAnglesUnits=rad  RotationMatrix=[1 0 0; 0 1 0; 0 0 1]
  iiwa_joint_1_AxisTransform : sm_lib/Frames and Transforms/Rigid Transform  TranslationMethod=Cartesian  TranslationStandardOffset=0  TranslationLengthUnit=m  TranslationStandardAxis=+Z  TranslationCartesianOffset=[0, 0, 0]  TranslationROffset=0  TranslationROffsetUnits=m  TranslationZOffset=0  TranslationZOffsetUnits=m  TranslationThetaOffset=0  TranslationThetaOffsetUnits=deg  RotationMethod=ArbitraryAxis  RotationAngleUnits=rad  RotationStandardAxis=+Z  RotationAngle=0  RotationArbitraryAxis=[1, 0, 0]  FollAlignAxisA=+X  BaseAlignAxisA=+Y  FollAlignAxisB=+Y  BaseAlignAxisB=+Z  RotationSequenceAxes=FollowerAxes  RotationSequence=XYX  RotationSequenceAngles=[0 0 0]  RotationSequenceAnglesUnits=deg  RotationMatrix=[1 0 0; 0 1 0; 0 0 1]
  iiwa_joint_1_OriginTransform : sm_lib/Frames and Transforms/Rigid Transform  TranslationMethod=Cartesian  TranslationStandardOffset=0  TranslationLengthUnit=m  TranslationStandardAxis=+Z  TranslationCartesianOffset=[0, 0, 0.15]  TranslationROffset=0  TranslationROffsetUnits=m  TranslationZOffset=0  TranslationZOffsetUnits=m  TranslationThetaOffset=0  TranslationThetaOffsetUnits=deg  RotationMethod=RotationSequence  RotationAngleUnits=deg  RotationStandardAxis=+Z  RotationAngle=0.0  RotationArbitraryAxis=[0 0 1]  FollAlignAxisA=+X  BaseAlignAxisA=+Y  FollAlignAxisB=+Y  BaseAlignAxisB=+Z  RotationSequenceAxes=BaseAxes  RotationSequence=XYZ  RotationSequenceAngles=[0, 0, 0]  RotationSequenceAnglesUnits=rad  RotationMatrix=[1 0 0; 0 1 0; 0 0 1]
  F : PMIOPort  Port=1  Side=Left
  F1 : PMIOPort  Port=2  Side=Right
  connections:
  Inertia/RConn1 -- InertiaOriginTransform/RConn1
  ReferenceFrame/RConn1 -- InertiaOriginTransform/LConn1 -- VisualOriginTransform/LConn1 -- iiwa_joint_1_OriginTransform/LConn1 -- F/RConn1
  Visual/RConn1 -- VisualOriginTransform/RConn1
  iiwa_joint_1_AxisTransform/RConn1 -- F1/RConn1
  iiwa_joint_1_AxisTransform/LConn1 -- iiwa_joint_1_OriginTransform/RConn1

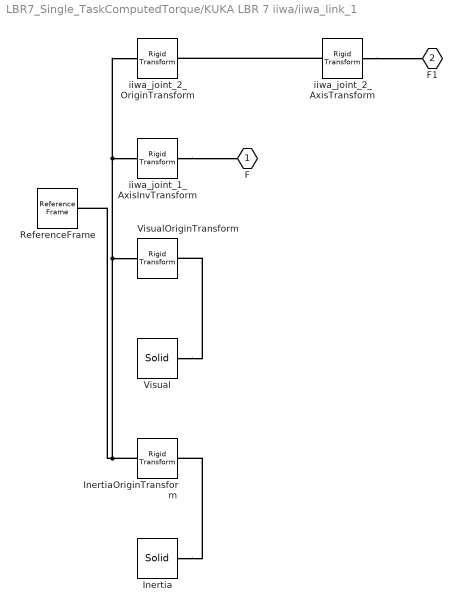
== system LBR7_Single_TaskComputedTorque/KUKA LBR 7 iiwa/iiwa_link_1 ==
  Inertia : sm_lib/Body Elements/Solid  InertiaType=Custom  Mass=3.4525  MassUnits=kg  CenterOfMass=[0, 0, 0]  CenterOfMassUnits=m  MomentsOfInertia=[0.02183, 0.007703, 0.02083]  MomentsOfInertiaUnits=kg*m^2  ProductsOfInertia=[0, 0, 0]  ProductsOfInertiaUnits=kg*m^2  DensityBased=on  Density=1000  DensityUnits=kg/m^3  DoExposeReferenceFrame=on  SerializedFrames=<Frames/>  GraphicType=None  MarkerShape=Sphere  MarkerSize=10  GraphicVisPropType=SimpleVisualProperties  GraphicDiffuseColor=[0.5 0.5 0.5]  GraphicSpecularColor=[0.5 0.5 0.5 1.0]  GraphicAmbientColor=[0.15 0.15 0.15 1.0]  GraphicEmissiveColor=[0.0 0.0 0.0 1.0]  GraphicShininess=75  GraphicOpacity=1.0  GeometryShape=Sphere  RectangleSize=[1 1]  RectangleSizeUnits=m  BrickDimensions=[1 1 1]  BrickDimensionUnits=m  CylinderRadius=1  CylinderRadiusUnits=m  CylinderLength=1  CylinderLengthUnits=m  SphereRadius=1  SphereRadiusUnits=m  EllipsoidRadii=[1 1 1]  EllipsoidRadiiUnits=m  ExtrusionCrossSection=[1 1; -1 1; -1 -1; 1 -1]  ExtrusionCrossSectionUnits=m  ExtrusionLength=1  ExtrusionLengthUnits=m  PolygonNumSides=3  PolygonOuterRadius=1  PolygonOuterRadiusUnits=m  ExtGeomFileType=STEP  ExtGeomFileUnits=m  RevolutionCrossSection=[1 1; 1 -1; 2 -1; 2 1]  RevolutionCrossSectionUnits=m  RevolutionExtent=Full  RevolutionAngle=180  RevolutionAngleUnits=deg
  InertiaOriginTransform : sm_lib/Frames and Transforms/Rigid Transform  TranslationMethod=Cartesian  TranslationStandardOffset=0  TranslationLengthUnit=m  TranslationStandardAxis=+Z  TranslationCartesianOffset=[0, -0.03, 0.12]  TranslationROffset=0  TranslationROffsetUnits=m  TranslationZOffset=0  TranslationZOffsetUnits=m  TranslationThetaOffset=0  TranslationThetaOffsetUnits=deg  RotationMethod=RotationSequence  RotationAngleUnits=deg  RotationStandardAxis=+Z  RotationAngle=0.0  RotationArbitraryAxis=[0 0 1]  FollAlignAxisA=+X  BaseAlignAxisA=+Y  FollAlignAxisB=+Y  BaseAlignAxisB=+Z  RotationSequenceAxes=BaseAxes  RotationSequence=XYZ  RotationSequenceAngles=[0, 0, 0]  RotationSequenceAnglesUnits=rad  RotationMatrix=[1 0 0; 0 1 0; 0 0 1]
  ReferenceFrame : sm_lib/Frames and Transforms/Reference Frame
  Visual : sm_lib/Body Elements/Solid  InertiaType=Custom  Mass=0  MassUnits=kg  CenterOfMass=[0, 0, 0]  CenterOfMassUnits=m  MomentsOfInertia=[0, 0, 0]  MomentsOfInertiaUnits=kg*m^2  ProductsOfInertia=[0, 0, 0]  ProductsOfInertiaUnits=kg*m^2  DensityBased=on  Density=1000  DensityUnits=kg/m^3  DoExposeReferenceFrame=on  SerializedFrames=<Frames/>  GraphicType=FromGeometry  MarkerShape=Sphere  MarkerSize=10  GraphicVisPropType=SimpleVisualProperties  GraphicDiffuseColor=[1, 0.423529411765, 0.0392156862745]  GraphicSpecularColor=[0.5 0.5 0.5 1.0]  GraphicAmbientColor=[0.15 0.15 0.15 1.0]  GraphicEmissiveColor=[0.0 0.0 0.0 1.0]  GraphicShininess=75  GraphicOpacity=1  GeometryShape=FromFile  RectangleSize=[1 1]  RectangleSizeUnits=m  BrickDimensions=[1 1 1]  BrickDimensionUnits=m  CylinderRadius=1  CylinderRadiusUnits=m  CylinderLength=1  CylinderLengthUnits=m  SphereRadius=1  SphereRadiusUnits=m  EllipsoidRadii=[1 1 1]  EllipsoidRadiiUnits=m  ExtrusionCrossSection=[1 1; -1 1; -1 -1; 1 -1]  ExtrusionCrossSectionUnits=m  ExtrusionLength=1  ExtrusionLengthUnits=m  PolygonNumSides=3  PolygonOuterRadius=1  PolygonOuterRadiusUnits=m  ExtGeomFileType=STL  ExtGeomFileName=link_1.stl  ExtGeomFileUnits=m  RevolutionCrossSection=[1 1; 1 -1; 2 -1; 2 1]  RevolutionCrossSectionUnits=m  RevolutionExtent=Full  RevolutionAngle=180  RevolutionAngleUnits=deg
  VisualOriginTransform : sm_lib/Frames and Transforms/Rigid Transform  TranslationMethod=Cartesian  TranslationStandardOffset=0  TranslationLengthUnit=m  TranslationStandardAxis=+Z  TranslationCartesianOffset=[0, 0, 0.0075]  TranslationROffset=0  TranslationROffsetUnits=m  TranslationZOffset=0  TranslationZOffsetUnits=m  TranslationThetaOffset=0  TranslationThetaOffsetUnits=deg  RotationMethod=RotationSequence  RotationAngleUnits=deg  RotationStandardAxis=+Z  RotationAngle=0.0  RotationArbitraryAxis=[0 0 1]  FollAlignAxisA=+X  BaseAlignAxisA=+Y  FollAlignAxisB=+Y  BaseAlignAxisB=+Z  RotationSequenceAxes=BaseAxes  RotationSequence=XYZ  RotationSequenceAngles=[0, 0, 0]  RotationSequenceAnglesUnits=rad  RotationMatrix=[1 0 0; 0 1 0; 0 0 1]
  iiwa_joint_1_AxisInvTransform : sm_lib/Frames and Transforms/Rigid Transform  TranslationMethod=Cartesian  TranslationStandardOffset=0  TranslationLengthUnit=m  TranslationStandardAxis=+Z  TranslationCartesianOffset=[0, 0, 0]  TranslationROffset=0  TranslationROffsetUnits=m  TranslationZOffset=0  TranslationZOffsetUnits=m  TranslationThetaOffset=0  TranslationThetaOffsetUnits=deg  RotationMethod=ArbitraryAxis  RotationAngleUnits=rad  RotationStandardAxis=+Z  RotationAngle=0  RotationArbitraryAxis=[1, 0, 0]  FollAlignAxisA=+X  BaseAlignAxisA=+Y  FollAlignAxisB=+Y  BaseAlignAxisB=+Z  RotationSequenceAxes=FollowerAxes  RotationSequence=XYX  RotationSequenceAngles=[0 0 0]  RotationSequenceAnglesUnits=deg  RotationMatrix=[1 0 0; 0 1 0; 0 0 1]
  iiwa_joint_2_AxisTransform : sm_lib/Frames and Transforms/Rigid Transform  TranslationMethod=Cartesian  TranslationStandardOffset=0  TranslationLengthUnit=m  TranslationStandardAxis=+Z  TranslationCartesianOffset=[0, 0, 0]  TranslationROffset=0  TranslationROffsetUnits=m  TranslationZOffset=0  TranslationZOffsetUnits=m  TranslationThetaOffset=0  TranslationThetaOffsetUnits=deg  RotationMethod=ArbitraryAxis  RotationAngleUnits=rad  RotationStandardAxis=+Z  RotationAngle=0  RotationArbitraryAxis=[1, 0, 0]  FollAlignAxisA=+X  BaseAlignAxisA=+Y  FollAlignAxisB=+Y  BaseAlignAxisB=+Z  RotationSequenceAxes=FollowerAxes  RotationSequence=XYX  RotationSequenceAngles=[0 0 0]  RotationSequenceAnglesUnits=deg  RotationMatrix=[1 0 0; 0 1 0; 0 0 1]
  iiwa_joint_2_OriginTransform : sm_lib/Frames and Transforms/Rigid Transform  TranslationMethod=Cartesian  TranslationStandardOffset=0  TranslationLengthUnit=m  TranslationStandardAxis=+Z  TranslationCartesianOffset=[0, 0, 0.19]  TranslationROffset=0  TranslationROffsetUnits=m  TranslationZOffset=0  TranslationZOffsetUnits=m  TranslationThetaOffset=0  TranslationThetaOffsetUnits=deg  RotationMethod=RotationSequence  RotationAngleUnits=deg  RotationStandardAxis=+Z  RotationAngle=0.0  RotationArbitraryAxis=[0 0 1]  FollAlignAxisA=+X  BaseAlignAxisA=+Y  FollAlignAxisB=+Y  BaseAlignAxisB=+Z  RotationSequenceAxes=BaseAxes  RotationSequence=XYZ  RotationSequenceAngles=[1.57079632679, 0, 3.14159265359]  RotationSequenceAnglesUnits=rad  RotationMatrix=[1 0 0; 0 1 0; 0 0 1]
  F : PMIOPort  Port=1  Side=Left
  F1 : PMIOPort  Port=2  Side=Right
  connections:
  Inertia/RConn1 -- InertiaOriginTransform/RConn1
  ReferenceFrame/RConn1 -- InertiaOriginTransform/LConn1 -- iiwa_joint_1_AxisInvTransform/LConn1 -- iiwa_joint_2_OriginTransform/LConn1 -- VisualOriginTransform/LConn1
  Visual/RConn1 -- VisualOriginTransform/RConn1
  iiwa_joint_1_AxisInvTransform/RConn1 -- F/RConn1
  iiwa_joint_2_AxisTransform/RConn1 -- F1/RConn1
  iiwa_joint_2_AxisTransform/LConn1 -- iiwa_joint_2_OriginTransform/RConn1

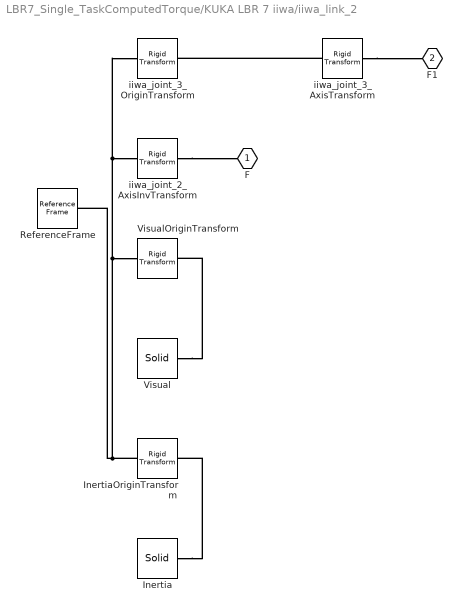
== system LBR7_Single_TaskComputedTorque/KUKA LBR 7 iiwa/iiwa_link_2 ==
  Inertia : sm_lib/Body Elements/Solid  InertiaType=Custom  Mass=3.4821  MassUnits=kg  CenterOfMass=[0, 0, 0]  CenterOfMassUnits=m  MomentsOfInertia=[0.02076, 0.02179, 0.00779]  MomentsOfInertiaUnits=kg*m^2  ProductsOfInertia=[0, 0, 0]  ProductsOfInertiaUnits=kg*m^2  DensityBased=on  Density=1000  DensityUnits=kg/m^3  DoExposeReferenceFrame=on  SerializedFrames=<Frames/>  GraphicType=None  MarkerShape=Sphere  MarkerSize=10  GraphicVisPropType=SimpleVisualProperties  GraphicDiffuseColor=[0.5 0.5 0.5]  GraphicSpecularColor=[0.5 0.5 0.5 1.0]  GraphicAmbientColor=[0.15 0.15 0.15 1.0]  GraphicEmissiveColor=[0.0 0.0 0.0 1.0]  GraphicShininess=75  GraphicOpacity=1.0  GeometryShape=Sphere  RectangleSize=[1 1]  RectangleSizeUnits=m  BrickDimensions=[1 1 1]  BrickDimensionUnits=m  CylinderRadius=1  CylinderRadiusUnits=m  CylinderLength=1  CylinderLengthUnits=m  SphereRadius=1  SphereRadiusUnits=m  EllipsoidRadii=[1 1 1]  EllipsoidRadiiUnits=m  ExtrusionCrossSection=[1 1; -1 1; -1 -1; 1 -1]  ExtrusionCrossSectionUnits=m  ExtrusionLength=1  ExtrusionLengthUnits=m  PolygonNumSides=3  PolygonOuterRadius=1  PolygonOuterRadiusUnits=m  ExtGeomFileType=STEP  ExtGeomFileUnits=m  RevolutionCrossSection=[1 1; 1 -1; 2 -1; 2 1]  RevolutionCrossSectionUnits=m  RevolutionExtent=Full  RevolutionAngle=180  RevolutionAngleUnits=deg
  InertiaOriginTransform : sm_lib/Frames and Transforms/Rigid Transform  TranslationMethod=Cartesian  TranslationStandardOffset=0  TranslationLengthUnit=m  TranslationStandardAxis=+Z  TranslationCartesianOffset=[0.0003, 0.059, 0.042]  TranslationROffset=0  TranslationROffsetUnits=m  TranslationZOffset=0  TranslationZOffsetUnits=m  TranslationThetaOffset=0  TranslationThetaOffsetUnits=deg  RotationMethod=RotationSequence  RotationAngleUnits=deg  RotationStandardAxis=+Z  RotationAngle=0.0  RotationArbitraryAxis=[0 0 1]  FollAlignAxisA=+X  BaseAlignAxisA=+Y  FollAlignAxisB=+Y  BaseAlignAxisB=+Z  RotationSequenceAxes=BaseAxes  RotationSequence=XYZ  RotationSequenceAngles=[0, 0, 0]  RotationSequenceAnglesUnits=rad  RotationMatrix=[1 0 0; 0 1 0; 0 0 1]
  ReferenceFrame : sm_lib/Frames and Transforms/Reference Frame
  Visual : sm_lib/Body Elements/Solid  InertiaType=Custom  Mass=0  MassUnits=kg  CenterOfMass=[0, 0, 0]  CenterOfMassUnits=m  MomentsOfInertia=[0, 0, 0]  MomentsOfInertiaUnits=kg*m^2  ProductsOfInertia=[0, 0, 0]  ProductsOfInertiaUnits=kg*m^2  DensityBased=on  Density=1000  DensityUnits=kg/m^3  DoExposeReferenceFrame=on  SerializedFrames=<Frames/>  GraphicType=FromGeometry  MarkerShape=Sphere  MarkerSize=10  GraphicVisPropType=SimpleVisualProperties  GraphicDiffuseColor=[1, 0.423529411765, 0.0392156862745]  GraphicSpecularColor=[0.5 0.5 0.5 1.0]  GraphicAmbientColor=[0.15 0.15 0.15 1.0]  GraphicEmissiveColor=[0.0 0.0 0.0 1.0]  GraphicShininess=75  GraphicOpacity=1  GeometryShape=FromFile  RectangleSize=[1 1]  RectangleSizeUnits=m  BrickDimensions=[1 1 1]  BrickDimensionUnits=m  CylinderRadius=1  CylinderRadiusUnits=m  CylinderLength=1  CylinderLengthUnits=m  SphereRadius=1  SphereRadiusUnits=m  EllipsoidRadii=[1 1 1]  EllipsoidRadiiUnits=m  ExtrusionCrossSection=[1 1; -1 1; -1 -1; 1 -1]  ExtrusionCrossSectionUnits=m  ExtrusionLength=1  ExtrusionLengthUnits=m  PolygonNumSides=3  PolygonOuterRadius=1  PolygonOuterRadiusUnits=m  ExtGeomFileType=STL  ExtGeomFileName=link_2.stl  ExtGeomFileUnits=m  RevolutionCrossSection=[1 1; 1 -1; 2 -1; 2 1]  RevolutionCrossSectionUnits=m  RevolutionExtent=Full  RevolutionAngle=180  RevolutionAngleUnits=deg
  VisualOriginTransform : sm_lib/Frames and Transforms/Rigid Transform  TranslationMethod=Cartesian  TranslationStandardOffset=0  TranslationLengthUnit=m  TranslationStandardAxis=+Z  TranslationCartesianOffset=[0, 0, 0]  TranslationROffset=0  TranslationROffsetUnits=m  TranslationZOffset=0  TranslationZOffsetUnits=m  TranslationThetaOffset=0  TranslationThetaOffsetUnits=deg  RotationMethod=RotationSequence  RotationAngleUnits=deg  RotationStandardAxis=+Z  RotationAngle=0.0  RotationArbitraryAxis=[0 0 1]  FollAlignAxisA=+X  BaseAlignAxisA=+Y  FollAlignAxisB=+Y  BaseAlignAxisB=+Z  RotationSequenceAxes=BaseAxes  RotationSequence=XYZ  RotationSequenceAngles=[0, 0, 0]  RotationSequenceAnglesUnits=rad  RotationMatrix=[1 0 0; 0 1 0; 0 0 1]
  iiwa_joint_2_AxisInvTransform : sm_lib/Frames and Transforms/Rigid Transform  TranslationMethod=Cartesian  TranslationStandardOffset=0  TranslationLengthUnit=m  TranslationStandardAxis=+Z  TranslationCartesianOffset=[0, 0, 0]  TranslationROffset=0  TranslationROffsetUnits=m  TranslationZOffset=0  TranslationZOffsetUnits=m  TranslationThetaOffset=0  TranslationThetaOffsetUnits=deg  RotationMethod=ArbitraryAxis  RotationAngleUnits=rad  RotationStandardAxis=+Z  RotationAngle=0  RotationArbitraryAxis=[1, 0, 0]  FollAlignAxisA=+X  BaseAlignAxisA=+Y  FollAlignAxisB=+Y  BaseAlignAxisB=+Z  RotationSequenceAxes=FollowerAxes  RotationSequence=XYX  RotationSequenceAngles=[0 0 0]  RotationSequenceAnglesUnits=deg  RotationMatrix=[1 0 0; 0 1 0; 0 0 1]
  iiwa_joint_3_AxisTransform : sm_lib/Frames and Transforms/Rigid Transform  TranslationMethod=Cartesian  TranslationStandardOffset=0  TranslationLengthUnit=m  TranslationStandardAxis=+Z  TranslationCartesianOffset=[0, 0, 0]  TranslationROffset=0  TranslationROffsetUnits=m  TranslationZOffset=0  TranslationZOffsetUnits=m  TranslationThetaOffset=0  TranslationThetaOffsetUnits=deg  RotationMethod=ArbitraryAxis  RotationAngleUnits=rad  RotationStandardAxis=+Z  RotationAngle=0  RotationArbitraryAxis=[1, 0, 0]  FollAlignAxisA=+X  BaseAlignAxisA=+Y  FollAlignAxisB=+Y  BaseAlignAxisB=+Z  RotationSequenceAxes=FollowerAxes  RotationSequence=XYX  RotationSequenceAngles=[0 0 0]  RotationSequenceAnglesUnits=deg  RotationMatrix=[1 0 0; 0 1 0; 0 0 1]
  iiwa_joint_3_OriginTransform : sm_lib/Frames and Transforms/Rigid Transform  TranslationMethod=Cartesian  TranslationStandardOffset=0  TranslationLengthUnit=m  TranslationStandardAxis=+Z  TranslationCartesianOffset=[0, 0.21, 0]  TranslationROffset=0  TranslationROffsetUnits=m  TranslationZOffset=0  TranslationZOffsetUnits=m  TranslationThetaOffset=0  TranslationThetaOffsetUnits=deg  RotationMethod=RotationSequence  RotationAngleUnits=deg  RotationStandardAxis=+Z  RotationAngle=0.0  RotationArbitraryAxis=[0 0 1]  FollAlignAxisA=+X  BaseAlignAxisA=+Y  FollAlignAxisB=+Y  BaseAlignAxisB=+Z  RotationSequenceAxes=BaseAxes  RotationSequence=XYZ  RotationSequenceAngles=[1.57079632679, 0, 3.14159265359]  RotationSequenceAnglesUnits=rad  RotationMatrix=[1 0 0; 0 1 0; 0 0 1]
  F : PMIOPort  Port=1  Side=Left
  F1 : PMIOPort  Port=2  Side=Right
  connections:
  Inertia/RConn1 -- InertiaOriginTransform/RConn1
  ReferenceFrame/RConn1 -- InertiaOriginTransform/LConn1 -- iiwa_joint_2_AxisInvTransform/LConn1 -- iiwa_joint_3_OriginTransform/LConn1 -- VisualOriginTransform/LConn1
  Visual/RConn1 -- VisualOriginTransform/RConn1
  iiwa_joint_2_AxisInvTransform/RConn1 -- F/RConn1
  iiwa_joint_3_AxisTransform/RConn1 -- F1/RConn1
  iiwa_joint_3_AxisTransform/LConn1 -- iiwa_joint_3_OriginTransform/RConn1
